simulink model "Manual_saturation_Block"  (R2024b)
settings: Solver=FixedStepAuto  StartTime=0.0  StopTime=10.0  FixedStep=0.0001  RelTol=1e-3
settings Model: Creator=abdal  LastModifiedBy=abdal

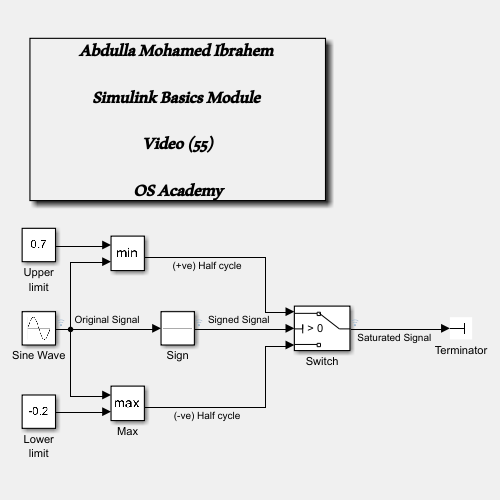
[thumbnail: Simulink's stored preview of the top-level diagram]
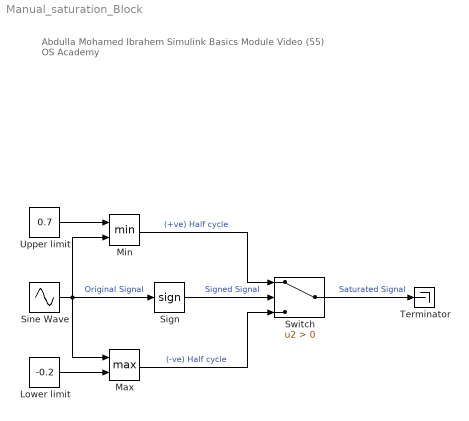
== system Manual_saturation_Block ==
  note: Abdulla Mohamed Ibrahem
      | Simulink Basics Module
      | Video (55)
      | OS Academy
  Lower limit : Constant  Value=-0.2
  Max : MinMax  Function=max  Inputs=2
  Min : MinMax  Inputs=2
  Sign : Signum
  Sine Wave : Sin  SampleTime=0
  Switch : Switch  Criteria=u2 > Threshold  SaturateOnIntegerOverflow=off  InputSameDT=off
  Terminator : Terminator
  Upper limit : Constant  Value=0.7
  wires:
  Sine Wave/1 -> Max/1, Min/2, Sign/1  "Original Signal"
  Sign/1 -> Switch/2  "Signed Signal"
  Upper limit/1 -> Min/1
  Min/1 -> Switch/1  "(+ve) Half cycle"
  Lower limit/1 -> Max/2
  Max/1 -> Switch/3  "(-ve) Half cycle"
  Switch/1 -> Terminator/1  "Saturated Signal"
